simulink model "Axis2DTest"  (R2016a)
settings: Solver=VariableStepAuto  StartTime=0.0  StopTime=11  RelTol=1e-3
libraries: SimscapeMacros x4, ProjectBlocks x3, fl_lib x1, nesl_utility x1, simulink x1
settings Model: Creator=Peter  LastModifiedBy=Peter

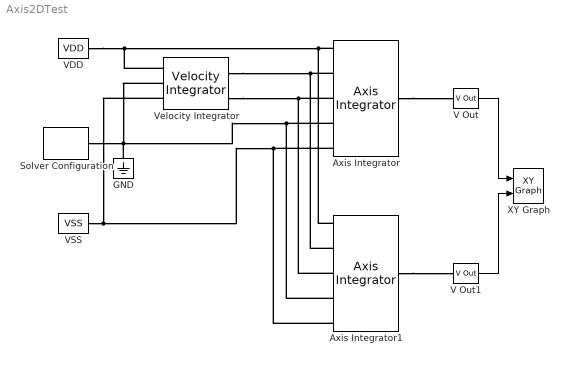
== system Axis2DTest ==
  Axis Integrator : ProjectBlocks/Axis Integrator
  Axis Integrator1 : ProjectBlocks/Axis Integrator
  GND : fl_lib/Electrical/Electrical Elements/Electrical Reference
  Solver Configuration : nesl_utility/Solver Configuration  PhysicalDomain=network_engine_domain  SubClassName=solver  LeftPortType=input  RightPortType=generic  Accelerate=off  Tones=[]  Harmonics=[]  SimulateNoise=off  Profile=off  UseLocalSampling=off  EnableSwitchedLinearOptims=on  FrequencyDomain=off  UseCCode=off  RelTol=0.001  AbsTol=1e-06  MinStep=1e-09  ToWorkspace=off  RevertToSquareIcSolve=off  NumHomotopyIterations=100  PhasorMode=off  PhasorModeNumHarmonics=1  OverrideAbsTol=off  DoDC=off  ResidualTolerance=1e-09  UseLocalSolver=off  LocalSolverChoice=NE_BACKWARD_EULER_ADVANCER  LocalSolverSampleTime=0.001  DoFixedCost=off  MaxNonlinIter=3  MaxModeIter=2  LinearAlgebra=Sparse  DelaysMemoryBudget=1024  AutomaticFiltering=on  FilteringTimeConstant=0.001
  V Out : SimscapeMacros/V Out
  V Out1 : SimscapeMacros/V Out
  VDD : SimscapeMacros/VDD
  VSS : SimscapeMacros/VSS
  Velocity Integrator : ProjectBlocks/Velocity Integrator
  XY Graph : simulink/Sinks/XY Graph  xmin=-5  xmax=5  ymin=-5  ymax=5  st=-1
  wires:
  V Out/1 -> XY Graph/1
  V Out1/1 -> XY Graph/2
  connections:
  VDD/RConn1 -- Velocity Integrator/LConn1 -- Axis Integrator1/LConn1 -- Axis Integrator/LConn1
  GND/LConn1 -- Solver Configuration/RConn1 -- Velocity Integrator/LConn2 -- Axis Integrator1/LConn4 -- Axis Integrator/LConn4
  VSS/RConn1 -- Velocity Integrator/LConn3 -- Axis Integrator1/LConn5 -- Axis Integrator/LConn5
  Velocity Integrator/RConn2 -- Axis Integrator1/LConn3 -- Axis Integrator/LConn3
  Axis Integrator/RConn1 -- V Out/LConn1
  Velocity Integrator/RConn1 -- Axis Integrator1/LConn2 -- Axis Integrator/LConn2
  Axis Integrator1/RConn1 -- V Out1/LConn1
